simulink model "question2_i"  (Simulink 7.1)
settings: Solver=ode45  StartTime=0.0  StopTime=10.0  RelTol=1e-3
settings Model: Creator=ALUNO  LastModifiedBy=ALUNO

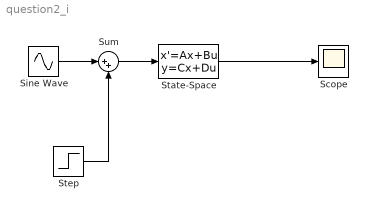
== system question2_i ==
  Scope : Scope
  Sine Wave : Sin  Frequency=5  SampleTime=0
  State-Space : StateSpace  A=-0.5  C=[0;1]  D=[2;0]
  Step : Step  Time=0  SampleTime=0
  Sum : Sum  Inputs=|++  OutDataType=sfix(16)  OutScaling=2^0
  wires:
  Sine Wave/1 -> Sum/1
  Sum/1 -> State-Space/1
  Step/1 -> Sum/2
  State-Space/1 -> Scope/1
